simulink model "windSimulation_2020a"  (R2020a)
settings: Solver=ode4  StartTime=0.0  StopTime=100  FixedStep=dt  RelTol=1e-3
values from neighbouring files (symbols this model uses):
  alt0 = 600    [initializeSim.m]
  dt = 0.1    [dryden_wind_model.m]    (also in filters.m; full_sim_and_filter_loop.m = 0.01; getDynamicsJacobian.m; initializeSim.m = 0.01)
  F = [0;0;0]    [simple_sim.m]
  gustWindFlag = 1    [initializeSim.m]
  initCovarianceEkf = diag([1e-3, 1e-3,                            2, 5e-3,                            1e-4, 1e-4,                            10, 10])    [initializeSim.m]
  initCovarianceUKF = diag([1e-3, 1e-3,                            2, 5e-3,                            1e-4, 1e-4,                            1, 1])    [initializeSim.m]
  initEstimateEkf = [0, 0,                     initGroundSpeedEst, initAttitude(3),                     windNorthStatic + 4*randn, windEastStatic + 4*randn,                     0, 0]    [initializeSim.m]
  initEstimateParticleFilter = [0, 0, initGroundSpeedEst, initAttitude(3), 15, -32]    [initializeSim.m]
  initEstimateUKF = [0, 0, initGroundSpeedEst, initAttitude(3),                    windNorthStatic + 1*randn, windEastStatic + 1*randn,                     0, 0]    [initializeSim.m]
  q = uKF(2)    [dynJacobian.m]    (also in getDynamicsJacobian.m; getDynamicsJacobianTest.m; getStateTransitionDynamics.m; simple_sim.m)
  Qekf = diag([1e-5, 1e-5,               1, 1e-3,               1, 1,               1, 1])    [initializeSim.m]
  Qukf = diag([1e-5, 1e-5,               1, 1e-3,               .1, .1,               .1, .1])    [initializeSim.m]
  r = uKF(3)    [dynJacobian.m]    (also in getDynamicsJacobian.m; getDynamicsJacobianTest.m; getStateTransitionDynamics.m; simple_sim.m)
  Rekf = diag([1, 1,               1, 1e-3,               1, 1])    [initializeSim.m]
  Rukf = diag([1, 1,               1, 1e-3,               1, 1])    [initializeSim.m]
  sensorNoiseFlag = 1    [initializeSim.m]
  staticWindFlag = 1    [initializeSim.m]
  turbulentWindFlag = 1    [initializeSim.m]
  var = getSensorVariances('low')    [getSensorVariances.m]    (also in initializeSim.m = getSensorVariances(suite))
  windDownStatic = 0    [initializeSim.m]
  windEastStatic = -9    [initializeSim.m]
  windNorthStatic = 14    [initializeSim.m]
undefined symbols (not defined in the file or in its folder): MIL, sigbuilder_block
libraries: aerolibwind2 x2, shared6dof x1, sharedtransform x1, aerolibasang x1, simulink_extras x1
settings Model: Creator=Don  LastModifiedBy=Somrita

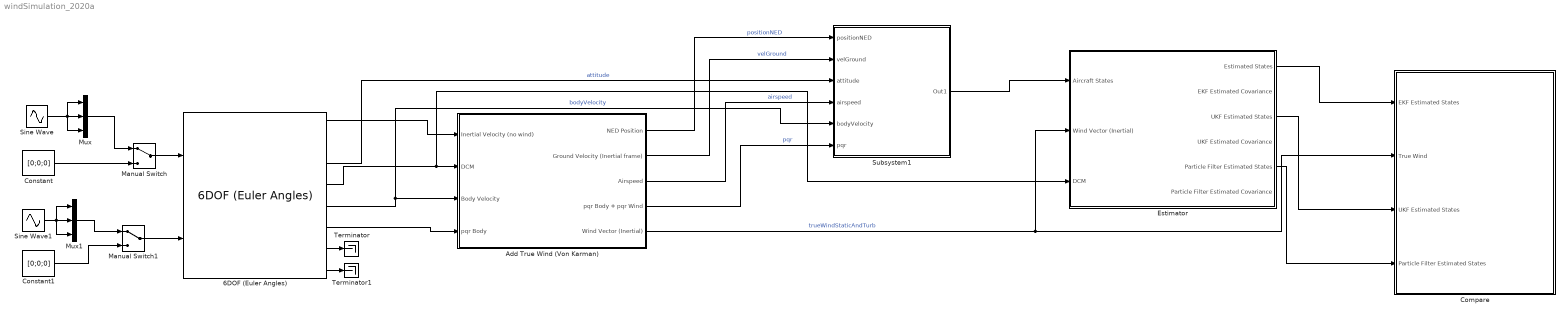
== system windSimulation_2020a ==
  6DOF (Euler Angles) : shared6dof/6DOF (Euler Angles)  units=Metric (MKS)  mtype=Fixed  rep=Euler Angles  xme_0=[0 0 -abs(alt0)]  Vm_0=initVelBody  eul_0=initAttitude  pm_0=[0 0 0]  mass_0=mass  mass_e=0.5  mass_f=2.0  inertia=J  inertia_e=eye(3)  inertia_f=2*eye(3)  k_quat=1.0  vre_flag=on  abi_flag=off  aMode=0  xme_statename=''  Vm_statename=''  eul_statename=''  quat_statename=''  pm_statename=''  mass_statename=''
      settings: SourceProductBaseCode=AE,PW,MT,UV,VE,VP
  Add True Wind (Von Karman) : Subsystem
  Compare : Subsystem
  Constant : Constant  Value=[0;0;0]
  Constant1 : Constant  Value=[0;0;0]
  Estimator : Subsystem
  Manual Switch : ManualSwitch
  Manual Switch1 : ManualSwitch
  Mux : Mux  Inputs=3
  Mux1 : Mux  Inputs=3
  Sine Wave : Sin  SampleTime=0
  Sine Wave1 : Sin  Amplitude=0.001  SampleTime=0
  Subsystem1 : Subsystem
  Terminator : Terminator
  Terminator1 : Terminator
  wires:
  Constant/1 -> Manual Switch/2
  Constant1/1 -> Manual Switch1/2
  6DOF (Euler Angles)/1 -> Add True Wind (Von Karman)/1(Inertial Velocity (no wind))
  6DOF (Euler Angles)/4 -> Estimator/3(DCM), Add True Wind (Von Karman)/2(DCM)
  6DOF (Euler Angles)/5 -> Add True Wind (Von Karman)/3(Body Velocity), Subsystem1/5(bodyVelocity)  "bodyVelocity"
  6DOF (Euler Angles)/6 -> Add True Wind (Von Karman)/4(pqr Body)
  Manual Switch/1 -> 6DOF (Euler Angles)/1
  Manual Switch1/1 -> 6DOF (Euler Angles)/2
  Sine Wave/1 -> Mux/2, Mux/1, Mux/3
  Mux/1 -> Manual Switch/1
  Sine Wave1/1 -> Mux1/2, Mux1/1, Mux1/3
  Mux1/1 -> Manual Switch1/1
  6DOF (Euler Angles)/7 -> Terminator/1
  6DOF (Euler Angles)/8 -> Terminator1/1
  Estimator/1(Estimated States) -> Compare/1(EKF Estimated States)
  Add True Wind (Von Karman)/5(Wind Vector (Inertial)) -> Estimator/2(Wind Vector (Inertial)), Compare/2(True Wind)  "trueWindStaticAndTurb"
  Estimator/3(UKF Estimated States) -> Compare/3(UKF Estimated States)
  Estimator/5(Particle Filter Estimated States) -> Compare/4(Particle Filter Estimated States)
  Add True Wind (Von Karman)/1(NED Position) -> Subsystem1/1(positionNED)  "positionNED"
  Add True Wind (Von Karman)/2(Ground Velocity (Inertial frame)) -> Subsystem1/2(velGround)  "velGround"
  6DOF (Euler Angles)/3 -> Subsystem1/3(attitude)  "attitude"
  Add True Wind (Von Karman)/3(Airspeed) -> Subsystem1/4(airspeed)  "airspeed"
  Add True Wind (Von Karman)/4(pqr Body + pqr Wind) -> Subsystem1/6(pqr)  "pqr"
  Subsystem1/1(Out1) -> Estimator/1(Aircraft States)

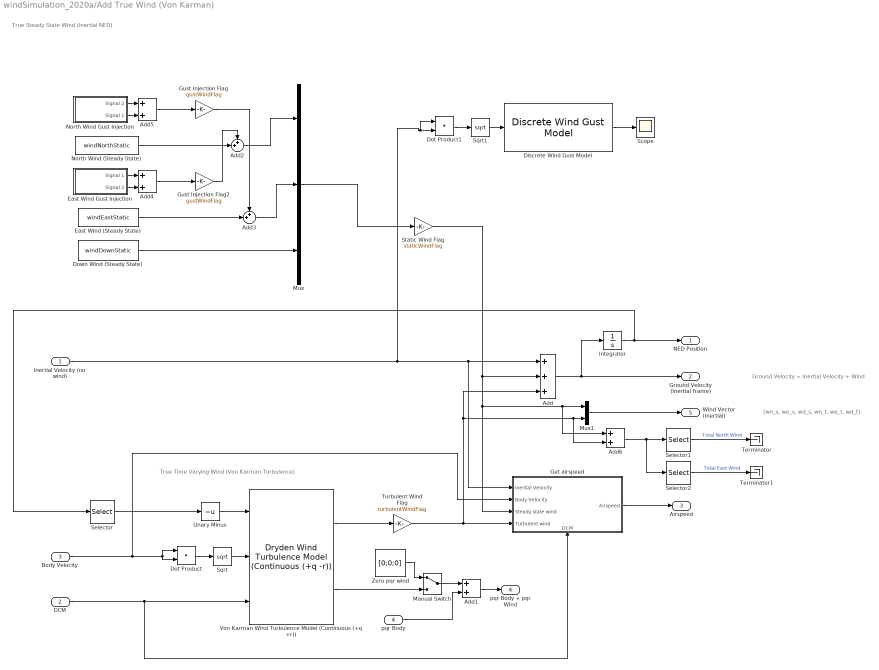
== system windSimulation_2020a/Add True Wind (Von Karman) ==
  note: [wn_s, we_s, wd_s, wn_t, we_t, wd_t]
  note: Ground Velocity = Inertial Velocity + Wind
  note: True Time Varying Wind (Von Karman Turbulence)
  note: True Steady State Wind (Inertial NED)
  Inertial Velocity (no wind) : Inport
  DCM : Inport  Port=2
  Body Velocity : Inport  Port=3
  pqr Body : Inport  Port=4
  Add : Sum  Inputs=+++
  Add{1,4..6} (4 alike) : Sum
  Add2 : Sum  Inputs=++|
  Add3 : Sum  Inputs=++|
  Discrete Wind Gust Model : aerolibwind2/Discrete Wind Gust Model  units=Metric (MKS)  Gx=on  Gy=on  Gz=on  t_0=5  d_m=[120 120 80]  v_m=[3.5 3.5 3.0]
  Dot Product : DotProduct  InputSameDT=on  OutDataTypeStr=Inherit: Inherit via internal rule
  Dot Product1 : DotProduct  InputSameDT=on  OutDataTypeStr=Inherit: Inherit via internal rule
  Down Wind (Steady State) : Constant  Value=windDownStatic
  East Wind (Steady State) : Constant  Value=windEastStatic
  East Wind Gust Injection : Subsystem  Tag=STV Subsys  LoadFcn=sigbuilder_block('load');  StartFcn=sigbuilder_block('start');  StopFcn=sigbuilder_block('stop');  ClipboardFcn=sigbuilder_block('clipboard');  mask(Sigbuilder block){tuvar=[0:10]}
      mask help: Simulink:masks:SigbuilderBlock_MD
      mask init:
      | if ~strcmp(get_param(bdroot(gcbh),'SimulationStatus'),'stopped') tuvar = sigbuilder_block('maskInit'); end
      settings: CopyFcn=sigbuilder_block('copy');  DeleteFcn=sigbuilder_block('delete');  ModelCloseFcn=sigbuilder_block('modelClose');  PreSaveFcn=sigbuilder_block('preSave');  PauseFcn=sigbuilder_block('pause');  ContinueFcn=sigbuilder_block('continue');  NameChangeFcn=sigbuilder_block('namechange');  OpenFcn=sigbuilder_block('open',[48.75 0 1391.25 750.75 ]);  CloseFcn=sigbuilder_block('close');
      mask Display: plot(0, 0, 100, 100,[2, 2, 32, 32, 2], [68, 8, 8, 68, 68],[32, 2], [38, 38], [32, 19, 2],[53, 60, 44], [32, 17, 17, 2],[16, 16, 31, 31]);txt = getActiveGroup(gcbh);text(2, 100, txt,'verticalAlignment', 'top');
  Get airspeed : Subsystem
      settings: PortSchema="{\"entries\":[{\"content\":{\"sides\":[{\"content\":{\"connectorIds\":[\"In1\",\"In2\",\"In3\",\"In4\"]},\"type\":\"ConnectorPlacement.EquallySpacedRectSide\",\"uuid\":\"813c2b5b-04f3-4ec3-a969-2504c20ca38b\"},{\"content\":{\"connectorIds\":[\"Out1\"],\"side\":\"RIGHT\"},\"type\":\"ConnectorPlacement.EquallySpacedRectSide\",\"uuid\":\"9f878792-4dd4-4000-acee-7f28349bdd5f\"},{\"content\":{\"connectorIds\":[],\"side\":\"TOP\"},\"type\":\"ConnectorPlacement.EquallySpacedRectSide\",\"uuid\":\"3d2ef613-18a7-4015-9ddb-8a03be605fb8\"},{\"content\":{\"connectorIds\":[\"In5\"],\"side\":\"BOTTOM\"},\"type\":\"ConnectorPlacement.EquallySpacedRectSide\",\"uuid\":\"121bcea6-4847-4a17-8a68-e62f0e126d50\"}]},\"type\":\"ConnectorPlacement.EquallySpacedConnector\",\"uuid\":\"0bfc4666-1d36-45c8-946f-537367ff2a54\"}],\"packageUris\":[\"http://schema.mathworks.com/mf0/Connector/19700101\"],\"version\":\"1.0\"}"
  Gust Injection Flag : Gain  Gain=gustWindFlag
  Gust Injection Flag2 : Gain  Gain=gustWindFlag
  Integrator : Integrator  InitialCondition=[0, 0, -abs(alt0)]
  Manual Switch : ManualSwitch
  Mux : Mux  Inputs=3
  Mux1 : Mux  Inputs=2
  North Wind (Steady State) : Constant  Value=windNorthStatic
  North Wind Gust Injection : Subsystem  Tag=STV Subsys  LoadFcn=sigbuilder_block('load');  StartFcn=sigbuilder_block('start');  StopFcn=sigbuilder_block('stop');  ClipboardFcn=sigbuilder_block('clipboard');  mask(Sigbuilder block){tuvar=[0:10]}
      mask help: Simulink:masks:SigbuilderBlock_MD
      mask init:
      | if ~strcmp(get_param(bdroot(gcbh),'SimulationStatus'),'stopped') tuvar = sigbuilder_block('maskInit'); end
      settings: CopyFcn=sigbuilder_block('copy');  DeleteFcn=sigbuilder_block('delete');  ModelCloseFcn=sigbuilder_block('modelClose');  PreSaveFcn=sigbuilder_block('preSave');  PauseFcn=sigbuilder_block('pause');  ContinueFcn=sigbuilder_block('continue');  NameChangeFcn=sigbuilder_block('namechange');  OpenFcn=sigbuilder_block('open',[48.75 0 1391.25 729.75 ]);  CloseFcn=sigbuilder_block('close');
      mask Display: plot(0, 0, 100, 100,[2, 2, 32, 32, 2], [68, 8, 8, 68, 68],[32, 2], [38, 38], [32, 19, 2],[53, 60, 44], [32, 17, 17, 2],[16, 16, 31, 31]);txt = getActiveGroup(gcbh);text(2, 100, txt,'verticalAlignment', 'top');
  Scope : Scope
  Selector : Selector  InputPortWidth=3  IndexOptions=Index vector (dialog)  Indices=3  OutputSizes=1
  Selector1 : Selector  InputPortWidth=3  IndexOptions=Index vector (dialog)  Indices=1  OutputSizes=1
  Selector2 : Selector  InputPortWidth=3  IndexOptions=Index vector (dialog)  Indices=2  OutputSizes=1
  Sqrt : Sqrt  SaturateOnIntegerOverflow=on
  Sqrt1 : Sqrt  SaturateOnIntegerOverflow=on
  Static Wind Flag : Gain  Gain=staticWindFlag
  Terminator : Terminator
  Terminator1 : Terminator
  Turbulent Wind Flag : Gain  Gain=turbulentWindFlag
  Unary Minus : UnaryMinus
  Von Karman Wind Turbulence Model (Continuous (+q +r)) : aerolibwind2/Dryden Wind Turbulence Model  (Continuous (+q -r))  units=Metric (MKS)  spec=MIL-F-8785C  model=Continuous Von Karman (+q +r)  W20=10  Wdeg=0  TurbProb=10^-1  L_high=762  Wingspan=10  ts=0.1  Seed=[23341 23342 23343 23344]  T_on=on
  Zero pqr wind : Constant  Value=[0;0;0]
  NED Position : Outport  PortDimensions=3
  Ground Velocity (Inertial frame) : Outport  Port=2
  Airspeed : Outport  Port=3  PortDimensions=1
  pqr Body + pqr Wind : Outport  Port=4
  Wind Vector (Inertial) : Outport  Port=5
  wires:
  Sqrt/1 -> Von Karman Wind Turbulence Model (Continuous (+q +r))/2
  Selector/1 -> Unary Minus/1
  Von Karman Wind Turbulence Model (Continuous (+q +r))/1 -> Turbulent Wind Flag/1
  Unary Minus/1 -> Von Karman Wind Turbulence Model (Continuous (+q +r))/1
  DCM/1 -> Get airspeed/5(DCM), Von Karman Wind Turbulence Model (Continuous (+q +r))/3
  Body Velocity/1 -> Get airspeed/2(Body Velocity), Dot Product/2, Dot Product/1
  Von Karman Wind Turbulence Model (Continuous (+q +r))/2 -> Manual Switch/2
  Add/1 -> Ground Velocity (Inertial frame)/1, Integrator/1
  Add1/1 -> pqr Body + pqr Wind/1
  pqr Body/1 -> Add1/2
  North Wind (Steady State)/1 -> Add2/2
  East Wind (Steady State)/1 -> Add3/2
  Down Wind (Steady State)/1 -> Mux/3
  Mux/1 -> Static Wind Flag/1
  Manual Switch/1 -> Add1/1
  Zero pqr wind/1 -> Manual Switch/1
  Get airspeed/1(Airspeed) -> Airspeed/1
  Dot Product/1 -> Sqrt/1
  Mux1/1 -> Wind Vector (Inertial)/1
  Integrator/1 -> Selector/1, NED Position/1
  Turbulent Wind Flag/1 -> Get airspeed/4(Turbulent wind), Add/3, Add6/2, Mux1/2
  Static Wind Flag/1 -> Add6/1, Mux1/1, Get airspeed/3(Steady state wind), Add/2
  Add3/1 -> Mux/2
  Add2/1 -> Mux/1
  East Wind Gust Injection/1(Signal 1) -> Add4/1
  East Wind Gust Injection/2(Signal 2) -> Add4/2
  Add4/1 -> Gust Injection Flag2/1
  Add5/1 -> Gust Injection Flag/1
  North Wind Gust Injection/1(Signal 2) -> Add5/1
  North Wind Gust Injection/2(Signal 1) -> Add5/2
  Gust Injection Flag/1 -> Add3/1
  Gust Injection Flag2/1 -> Add2/1
  Sqrt1/1 -> Discrete Wind Gust Model/1
  Dot Product1/1 -> Sqrt1/1
  Inertial Velocity (no wind)/1 -> Dot Product1/1, Dot Product1/2, Get airspeed/1(Inertial Velocity), Add/1
  Discrete Wind Gust Model/1 -> Scope/1
  Add6/1 -> Selector2/1, Selector1/1
  Selector1/1 -> Terminator/1  "Total North Wind"
  Selector2/1 -> Terminator1/1  "Total East Wind"

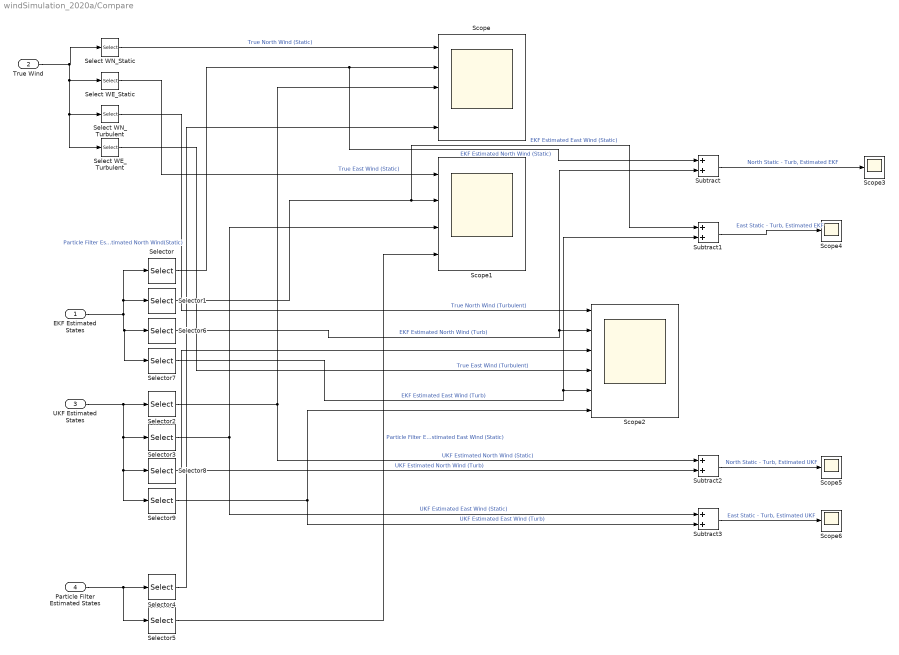
== system windSimulation_2020a/Compare ==
  EKF Estimated States : Inport
  True Wind : Inport  Port=2
  UKF Estimated States : Inport  Port=3
  Particle Filter Estimated States : Inport  Port=4
  Scope : Scope  NumInputPorts=5
  Scope1 : Scope  NumInputPorts=4
  Scope2 : Scope  NumInputPorts=6
  Scope{3..6} (4 alike) : Scope
  Select WE_Static : Selector  InputPortWidth=6  IndexOptions=Index vector (dialog)  Indices=2  OutputSizes=1
  Select WE_Turbulent : Selector  InputPortWidth=6  IndexOptions=Index vector (dialog)  Indices=5  OutputSizes=1
  Select WN_Static : Selector  InputPortWidth=6  IndexOptions=Index vector (dialog)  Indices=1  OutputSizes=1
  Select WN_Turbulent : Selector  InputPortWidth=6  IndexOptions=Index vector (dialog)  Indices=4  OutputSizes=1
  Selector : Selector  InputPortWidth=nEstStates  IndexOptions=Index vector (dialog)  Indices=5  OutputSizes=1
  Selector1 : Selector  InputPortWidth=nEstStates  IndexOptions=Index vector (dialog)  Indices=6  OutputSizes=1
  Selector2 : Selector  InputPortWidth=nEstStates  IndexOptions=Index vector (dialog)  Indices=5  OutputSizes=1
  Selector3 : Selector  InputPortWidth=nEstStates  IndexOptions=Index vector (dialog)  Indices=6  OutputSizes=1
  Selector4 : Selector  InputPortWidth=nEstStates  IndexOptions=Index vector (dialog)  Indices=5  OutputSizes=1
  Selector5 : Selector  InputPortWidth=nEstStates  IndexOptions=Index vector (dialog)  Indices=6  OutputSizes=1
  Selector6 : Selector  InputPortWidth=nEstStates  IndexOptions=Index vector (dialog)  Indices=7  OutputSizes=1
  Selector7 : Selector  InputPortWidth=nEstStates  IndexOptions=Index vector (dialog)  Indices=8  OutputSizes=1
  Selector8 : Selector  InputPortWidth=nEstStates  IndexOptions=Index vector (dialog)  Indices=7  OutputSizes=1
  Selector9 : Selector  InputPortWidth=nEstStates  IndexOptions=Index vector (dialog)  Indices=8  OutputSizes=1
  Subtract{,1..3} (4 alike) : Sum
  wires:
  EKF Estimated States/1 -> Selector7/1, Selector6/1, Selector1/1, Selector/1
  True Wind/1 -> Select WE_Turbulent/1, Select WN_Turbulent/1, Select WE_Static/1, Select WN_Static/1
  Selector/1 -> Subtract/1, Scope/2  "EKF Estimated North Wind (Static)"
  Select WN_Static/1 -> Scope/1  "True North Wind (Static)"
  Selector1/1 -> Subtract1/1, Scope1/2  "EKF Estimated East Wind (Static)"
  Select WE_Static/1 -> Scope1/1  "True East Wind (Static)"
  UKF Estimated States/1 -> Selector9/1, Selector8/1, Selector3/1, Selector2/1
  Selector2/1 -> Scope/3, Subtract2/1  "UKF Estimated North Wind (Static)"
  Selector3/1 -> Scope1/3, Subtract3/1  "UKF Estimated East Wind (Static)"
  Particle Filter Estimated States/1 -> Selector5/1, Selector4/1
  Selector4/1 -> Scope/5  "Particle Filter Estimated North Wind(Static)"
  Selector5/1 -> Scope1/4  "Particle Filter Estimated East Wind (Static)"
  Selector6/1 -> Subtract/2, Scope2/2  "EKF Estimated North Wind (Turb)"
  Selector7/1 -> Subtract1/2, Scope2/5  "EKF Estimated East Wind (Turb)"
  Select WN_Turbulent/1 -> Scope2/1  "True North Wind (Turbulent)"
  Select WE_Turbulent/1 -> Scope2/4  "True East Wind (Turbulent)"
  Subtract/1 -> Scope3/1  "North Static - Turb, Estimated EKF"
  Subtract1/1 -> Scope4/1  "East Static - Turb, Estimated EKF"
  Selector8/1 -> Subtract2/2, Scope2/3  "UKF Estimated North Wind (Turb)"
  Selector9/1 -> Subtract3/2, Scope2/6  "UKF Estimated East Wind (Turb)"
  Subtract3/1 -> Scope6/1  "East Static - Turb, Estimated UKF"
  Subtract2/1 -> Scope5/1  "North Static - Turb, Estimated UKF"

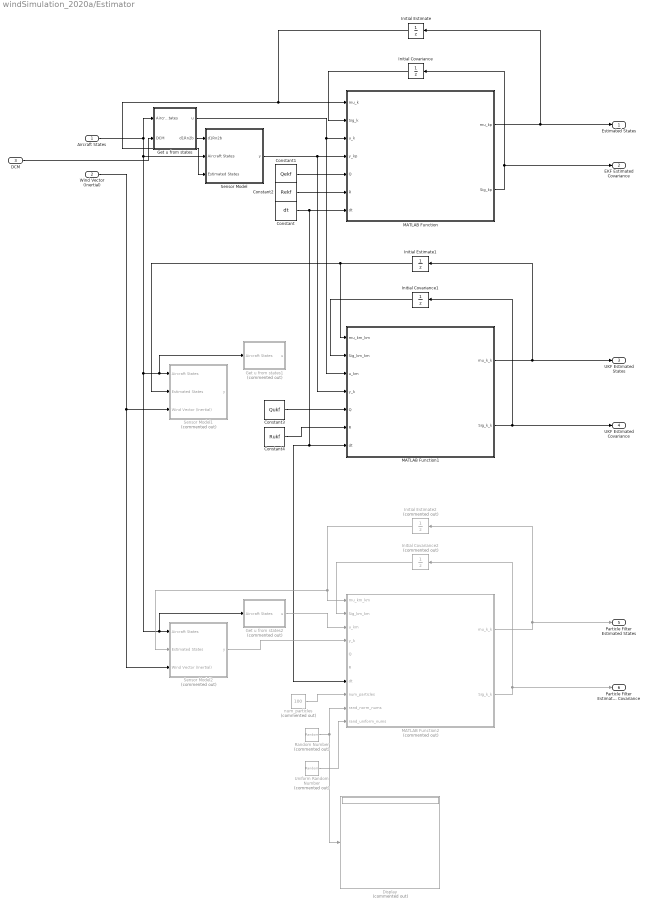
== system windSimulation_2020a/Estimator ==
  Aircraft States : Inport
  Wind Vector (Inertial) : Inport  Port=2
  DCM : Inport  Port=3
  Constant : Constant  Value=dt
  Constant1 : Constant  Value=Qekf
  Constant2 : Constant  Value=Rekf
  Constant3 : Constant  Value=Qukf
  Constant4 : Constant  Value=Rukf
  Display : Display  Commented=on
  Get u from states : Subsystem
  Get u from states1 : Subsystem  Commented=on
  Get u from states2 : Subsystem  Commented=on
  Initial Covariance : UnitDelay  InitialCondition=initCovarianceEkf  SampleTime=-1  HasFrameUpgradeWarning=on
  Initial Covariance1 : UnitDelay  InitialCondition=initCovarianceUKF  SampleTime=-1  HasFrameUpgradeWarning=on
  Initial Covariance2 : UnitDelay  Commented=on  InitialCondition=initCovarianceEkf  SampleTime=-1  HasFrameUpgradeWarning=on
  Initial Estimate : UnitDelay  InitialCondition=initEstimateEkf  SampleTime=-1  HasFrameUpgradeWarning=on
  Initial Estimate1 : UnitDelay  InitialCondition=initEstimateUKF  SampleTime=-1  HasFrameUpgradeWarning=on
  Initial Estimate2 : UnitDelay  Commented=on  InitialCondition=initEstimateParticleFilter  SampleTime=-1  HasFrameUpgradeWarning=on
  MATLAB Function : MATLAB Function  TreatAsAtomicUnit=on
  MATLAB Function1 : MATLAB Function  TreatAsAtomicUnit=on
  MATLAB Function2 : MATLAB Function  Commented=on  TreatAsAtomicUnit=on
  Random Number : RandomNumber  Commented=on  Mean=zeros(100*6,1)  Seed=1:6*100  SampleTime=0.1
  Sensor Model : Subsystem
  Sensor Model1 : Subsystem  Commented=on
  Sensor Model2 : Subsystem  Commented=on
  Uniform Random Number : UniformRandomNumber  Commented=on  Minimum=zeros(100,1)  Maximum=ones(100,1)  Seed=1:100  SampleTime=0.1
  num_particles : Constant  Commented=on  Value=100
  Estimated States : Outport
  EKF Estimated Covariance : Outport  Port=2
  UKF Estimated States : Outport  Port=3
  UKF Estimated Covariance : Outport  Port=4
  Particle Filter Estimated States : Outport  Port=5
  Particle Filter Estimated Covariance : Outport  Port=6
  wires:
  MATLAB Function/1(mu_kp) -> Initial Estimate/1, Estimated States/1
  Initial Estimate/1 -> Sensor Model/3(Estimated States), MATLAB Function/1(mu_k)
  MATLAB Function/2(Sig_kp) -> EKF Estimated Covariance/1, Initial Covariance/1
  Initial Covariance/1 -> MATLAB Function/2(Sig_k)
  MATLAB Function1/1(mu_k_k) -> UKF Estimated States/1, Initial Estimate1/1
  MATLAB Function1/2(Sig_k_k) -> UKF Estimated Covariance/1, Initial Covariance1/1
  Initial Estimate1/1 -> MATLAB Function1/1(mu_km_km), Sensor Model1/2(Estimated States)
  Initial Covariance1/1 -> MATLAB Function1/2(Sig_km_km)
  MATLAB Function2/1(mu_k_k) -> Particle Filter Estimated States/1, Initial Estimate2/1
  Constant/1 -> MATLAB Function2/7(dt), MATLAB Function1/7(dt), MATLAB Function/7(dt)
  Sensor Model/1(y) -> MATLAB Function1/4(y_k), MATLAB Function/4(y_kp)
  MATLAB Function2/2(Sig_k_k) -> Particle Filter Estimated Covariance/1, Initial Covariance2/1
  Constant2/1 -> MATLAB Function/6(R)
  Constant1/1 -> MATLAB Function/5(Q)
  Initial Covariance2/1 -> MATLAB Function2/2(Sig_km_km)
  Get u from states/1(u) -> MATLAB Function1/3(u_km), MATLAB Function/3(u_k)
  Random Number/1 -> Display/1, MATLAB Function2/9(rand_norm_nums)
  num_particles/1 -> MATLAB Function2/8(num_particles)
  Uniform Random Number/1 -> MATLAB Function2/10(rand_uniform_nums)
  Wind Vector (Inertial)/1 -> Sensor Model2/3(Wind Vector (Inertial)), Sensor Model1/3(Wind Vector (Inertial))
  Aircraft States/1 -> Sensor Model2/1(Aircraft States), Get u from states2/1(Aircraft States), Sensor Model1/1(Aircraft States), Get u from states1/1(Aircraft States), Sensor Model/2(Aircraft States), Get u from states/1(Aircraft States)
  Initial Estimate2/1 -> MATLAB Function2/1(mu_km_km), Sensor Model2/2(Estimated States)
  Get u from states2/1(u) -> MATLAB Function2/3(u_km)
  Sensor Model2/1(y) -> MATLAB Function2/4(y_k)
  Constant3/1 -> MATLAB Function1/5(Q)
  Constant4/1 -> MATLAB Function1/6(R)
  Get u from states/2(d1Rn2b) -> Sensor Model/1(d1Rn2b)
  DCM/1 -> Get u from states/2(DCM)

== system windSimulation_2020a/Subsystem1 ==
  note: xyzInertial, uvwGround, attitude, pqr, airspeed, groundSpeed, courseAngle
  positionNED : Inport
  velGround : Inport  Port=2
  attitude : Inport  Port=3
  airspeed : Inport  Port=4
  bodyVelocity : Inport  Port=5
  pqr : Inport  Port=6
  Get ground speed and course angle : Subsystem
  Mux2 : Mux  Inputs=8
  Subsystem : Subsystem
  Out1 : Outport
  wires:
  positionNED/1 -> Mux2/1
  airspeed/1 -> Mux2/5
  Subsystem/1(Aligned Attitude) -> Mux2/3
  bodyVelocity/1 -> Mux2/8, Subsystem/2(bodyVelocity)
  attitude/1 -> Subsystem/1(Attitude)
  Get ground speed and course angle/1(Ground Speed) -> Mux2/6  "trueGroundspeed"
  Get ground speed and course angle/2(Course Angle) -> Mux2/7  "trueCourseAngle"
  velGround/1 -> Mux2/2, Get ground speed and course angle/1(Ground Velocity)
  Mux2/1 -> Out1/1
  pqr/1 -> Mux2/4

== system windSimulation_2020a/Add True Wind (Von Karman)/East Wind Gust Injection ==
  Demux : Demux  Tag=STV Demux  Outputs=2
      settings: DisplayOption=none
  FromWs : FromWorkspace  Tag=STV FromWs  VariableName=tuvar
      SigBuilderData=|
      | common.afterFinalStr = 'Extrapolate'
      | common.sampleTime = 0
      | dataSet.timeRange = [0 100]
      | dataSet.name = 'Group 1'
      | sbobj.Groups.Name = 'Group 1'
      | sbobj.Groups.Signals(1).Name = 'Signal 1'
      | sbobj.Groups.Signals(1).XData = [0 6 6 18 18 100]
      | sbobj.Groups.Signals(1).YData = [0 0 7 7 0 0]
      | sbobj.Groups.Signals(2).Name = 'Signal 2'
      | sbobj.Groups.Signals(2).XData = [0 42 42 58 58 100]
      | sbobj.Groups.Signals(2).YData = [0 0 -3 -3 0 0]
      | sbobj.Groups.TimeRange = [0 100]
  Signal 1 : Outport  Tag=STV Outport
  Signal 2 : Outport  Tag=STV Outport  Port=2
  wires:
  FromWs/1 -> Demux/1
  Demux/1 -> Signal 1/1
  Demux/2 -> Signal 2/1

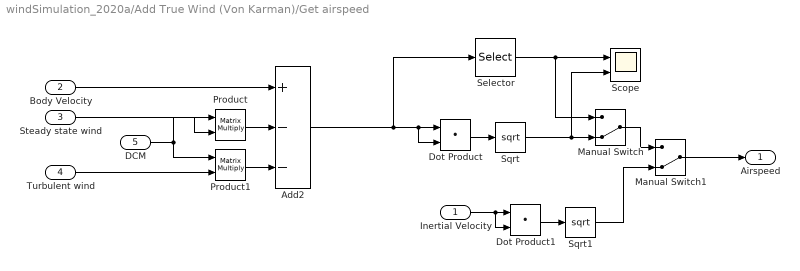
== system windSimulation_2020a/Add True Wind (Von Karman)/Get airspeed ==
  Inertial Velocity : Inport
  Body Velocity : Inport  Port=2
  Steady state wind : Inport  Port=3
  Turbulent wind : Inport  Port=4
  DCM : Inport  Port=5
  Add2 : Sum  Inputs=+--
  Dot Product : DotProduct  InputSameDT=on  OutDataTypeStr=Inherit: Inherit via internal rule
  Dot Product1 : DotProduct  InputSameDT=on  OutDataTypeStr=Inherit: Inherit via internal rule
  Manual Switch : ManualSwitch  CurrentSetting=0
  Manual Switch1 : ManualSwitch  CurrentSetting=0
  Product : Product  Multiplication=Matrix(*)
  Product1 : Product  Multiplication=Matrix(*)
  Scope : Scope  NumInputPorts=2
  Selector : Selector  InputPortWidth=3  IndexOptions=Index vector (dialog)  Indices=1  OutputSizes=1
  Sqrt : Sqrt  SaturateOnIntegerOverflow=on
  Sqrt1 : Sqrt  SaturateOnIntegerOverflow=on
  Airspeed : Outport
  wires:
  Body Velocity/1 -> Add2/1
  Steady state wind/1 -> Product/2
  Add2/1 -> Dot Product/2, Dot Product/1, Selector/1
  Turbulent wind/1 -> Product1/2
  DCM/1 -> Product/1, Product1/1
  Product/1 -> Add2/2
  Product1/1 -> Add2/3
  Manual Switch/1 -> Manual Switch1/1
  Selector/1 -> Manual Switch/1, Scope/1
  Dot Product/1 -> Sqrt/1
  Sqrt/1 -> Scope/2, Manual Switch/2
  Manual Switch1/1 -> Airspeed/1
  Dot Product1/1 -> Sqrt1/1
  Inertial Velocity/1 -> Dot Product1/1, Dot Product1/2
  Sqrt1/1 -> Manual Switch1/2

== system windSimulation_2020a/Add True Wind (Von Karman)/North Wind Gust Injection ==
  Demux : Demux  Tag=STV Demux  Outputs=2
      settings: DisplayOption=none
  FromWs : FromWorkspace  Tag=STV FromWs  VariableName=tuvar
      SigBuilderData=|
      | common.afterFinalStr = 'Extrapolate'
      | common.sampleTime = 0
      | dataSet.timeRange = [0 100]
      | dataSet.name = 'Group 1'
      | sbobj.Groups.Name = 'Group 1'
      | sbobj.Groups.Signals(1).Name = 'Signal 2'
      | sbobj.Groups.Signals(1).XData = [0 52 52 69 69.1 100]
      | sbobj.Groups.Signals(1).YData = [0 0 6 6 0 0]
      | sbobj.Groups.Signals(2).Name = 'Signal 1'
      | sbobj.Groups.Signals(2).XData = [0 8 8 23 23 100]
      | sbobj.Groups.Signals(2).YData = [0 0 -4 -4 0 0]
      | sbobj.Groups.TimeRange = [0 100]
  Signal 2 : Outport  Tag=STV Outport
  Signal 1 : Outport  Tag=STV Outport  Port=2
  wires:
  FromWs/1 -> Demux/1
  Demux/1 -> Signal 2/1
  Demux/2 -> Signal 1/1

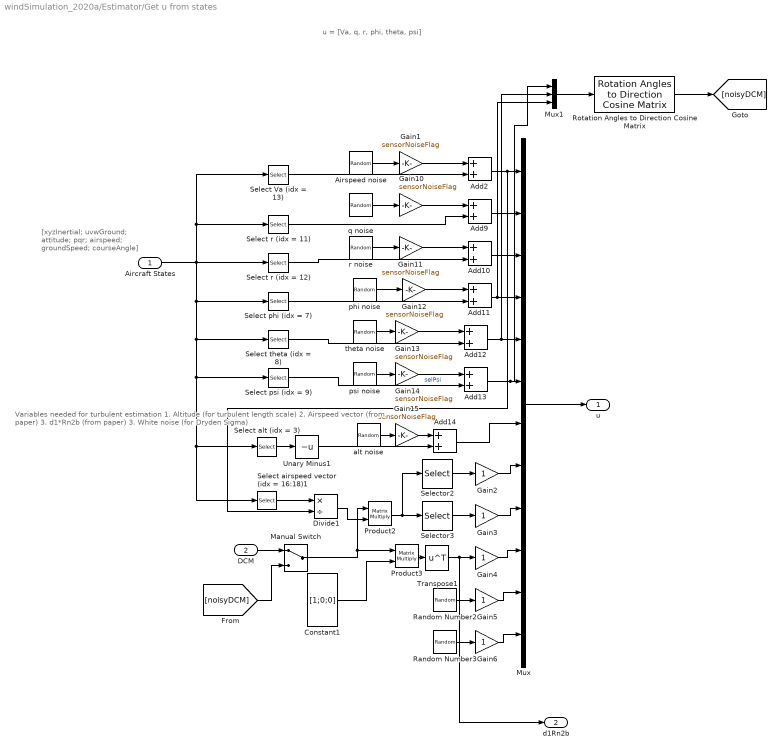
== system windSimulation_2020a/Estimator/Get u from states ==
  note: Variables needed for turbulent estimation
      | 	1. Altitude (for turbulent length scale)
      | 	2. Airspeed vector (from paper)
      | 	3. d1*Rn2b (from paper)
      | 	3. White noise (for Dryden Sigma)
  note: u = [Va, q, r, phi, theta, psi]
  note: [xyzInertial;
      | uvwGround;
      | attitude;
      | pqr;
      | airspeed;
      | groundSpeed;
      | courseAngle]
  Aircraft States : Inport
  DCM : Inport  Port=2
  Add{2,9..14} (7 alike) : Sum
  Airspeed noise : RandomNumber  Variance=var.airspeed_mps  SampleTime=dt
  Constant1 : Constant  Value=[1;0;0]  VectorParams1D=off
  Divide1 : Product  Inputs=*/
  Gain{1,10..15} (7 alike) : Gain  Gain=sensorNoiseFlag
  Gain{2..6} (5 alike) : Gain
  Manual Switch : ManualSwitch
  Mux : Mux  Inputs=12
  Mux1 : Mux  Inputs=3
  Product2 : Product  Multiplication=Matrix(*)
  Product3 : Product  Multiplication=Matrix(*)
  Random Number2 : RandomNumber  SampleTime=dt
  Random Number3 : RandomNumber  Seed=100  SampleTime=dt
  Rotation Angles to Direction Cosine Matrix : sharedtransform/Rotation Angles to Direction Cosine Matrix  rotationOrder=ZYX  aMode=aMode
      settings: SourceProductBaseCode=AE,PW,MT,UV,VE,VP
  Select Va (idx = 13) : Selector  InputPortWidth=nStates  IndexOptions=Index vector (dialog)  Indices=13  OutputSizes=1
  Select airspeed vector (idx = 16:18)1 : Selector  InputPortWidth=nStates  IndexOptions=Index vector (dialog)  Indices=[16:18]  OutputSizes=1
  Select alt (idx = 3) : Selector  InputPortWidth=nStates  IndexOptions=Index vector (dialog)  Indices=3  OutputSizes=1
  Select phi (idx = 7) : Selector  InputPortWidth=nStates  IndexOptions=Index vector (dialog)  Indices=7  OutputSizes=1
  Select psi (idx = 9) : Selector  InputPortWidth=nStates  IndexOptions=Index vector (dialog)  Indices=9  OutputSizes=1
  Select r (idx = 11) : Selector  InputPortWidth=nStates  IndexOptions=Index vector (dialog)  Indices=11  OutputSizes=1
  Select r (idx = 12) : Selector  InputPortWidth=nStates  IndexOptions=Index vector (dialog)  Indices=12  OutputSizes=1
  Select theta (idx = 8) : Selector  InputPortWidth=nStates  IndexOptions=Index vector (dialog)  Indices=8  OutputSizes=1
  Selector2 : Selector  InputPortWidth=3  IndexOptions=Index vector (dialog)  Indices=1  OutputSizes=1
  Selector3 : Selector  InputPortWidth=3  IndexOptions=Index vector (dialog)  Indices=2  OutputSizes=1
  Transpose1 : Math  Operator=transpose  SaturateOnIntegerOverflow=on
  Unary Minus1 : UnaryMinus
  alt noise : RandomNumber  Variance=var.altitude_m  SampleTime=dt
  phi noise : RandomNumber  Variance=var.attitude_rad  SampleTime=dt
  psi noise : RandomNumber  Variance=var.attitude_rad * 3  SampleTime=dt
  q noise : RandomNumber  Variance=var.pqr_radps  SampleTime=dt
  r noise : RandomNumber  Variance=var.pqr_radps  SampleTime=dt
  theta noise : RandomNumber  Variance=var.attitude_rad  SampleTime=dt
  u : Outport
  d1Rn2b : Outport  Port=2
  wires:
  Aircraft States/1 -> Select airspeed vector (idx = 16:18)1/1, Select alt (idx = 3)/1, Select psi (idx = 9)/1, Select theta (idx = 8)/1, Select phi (idx = 7)/1, Select r (idx = 12)/1, Select r (idx = 11)/1, Select Va (idx = 13)/1
  Mux/1 -> u/1
  Select Va (idx = 13)/1 -> Add2/2
  Gain1/1 -> Add2/1
  Airspeed noise/1 -> Gain1/1
  Add2/1 -> Divide1/2, Mux/1
  q noise/1 -> Gain10/1
  Gain15/1 -> Add14/1
  Add9/1 -> Mux/2
  Add11/1 -> Mux1/3, Mux/4
  Add13/1 -> Mux1/1, Mux/6
  Add12/1 -> Mux1/2, Mux/5
  alt noise/1 -> Gain15/1
  Gain14/1 -> Add13/1
  theta noise/1 -> Gain13/1
  Add10/1 -> Mux/3
  r noise/1 -> Gain11/1
  Gain12/1 -> Add11/1
  Gain11/1 -> Add10/1
  psi noise/1 -> Gain14/1
  Gain13/1 -> Add12/1
  Gain10/1 -> Add9/1
  phi noise/1 -> Gain12/1
  Select r (idx = 11)/1 -> Add9/2
  Select r (idx = 12)/1 -> Add10/2
  Select phi (idx = 7)/1 -> Add11/2
  Select theta (idx = 8)/1 -> Add12/2
  Select psi (idx = 9)/1 -> Add13/2  "selPsi"
  Select alt (idx = 3)/1 -> Unary Minus1/1
  Unary Minus1/1 -> Add14/2
  Select airspeed vector (idx = 16:18)1/1 -> Divide1/1
  Divide1/1 -> Product2/2
  Selector2/1 -> Gain2/1
  Selector3/1 -> Gain3/1
  Product2/1 -> Selector2/1, Selector3/1
  Gain2/1 -> Mux/8
  Gain3/1 -> Mux/9
  Transpose1/1 -> d1Rn2b/1, Gain4/1
  Product3/1 -> Transpose1/1
  Constant1/1 -> Product3/2
  Random Number2/1 -> Gain5/1
  Random Number3/1 -> Gain6/1
  Gain4/1 -> Mux/10
  Gain5/1 -> Mux/11
  Gain6/1 -> Mux/12
  Add14/1 -> Mux/7
  Mux1/1 -> Rotation Angles to Direction Cosine Matrix/1
  Rotation Angles to Direction Cosine Matrix/1 -> [noisyDCM]
  [noisyDCM] -> Manual Switch/2
  Manual Switch/1 -> Product2/1, Product3/1
  DCM/1 -> Manual Switch/1

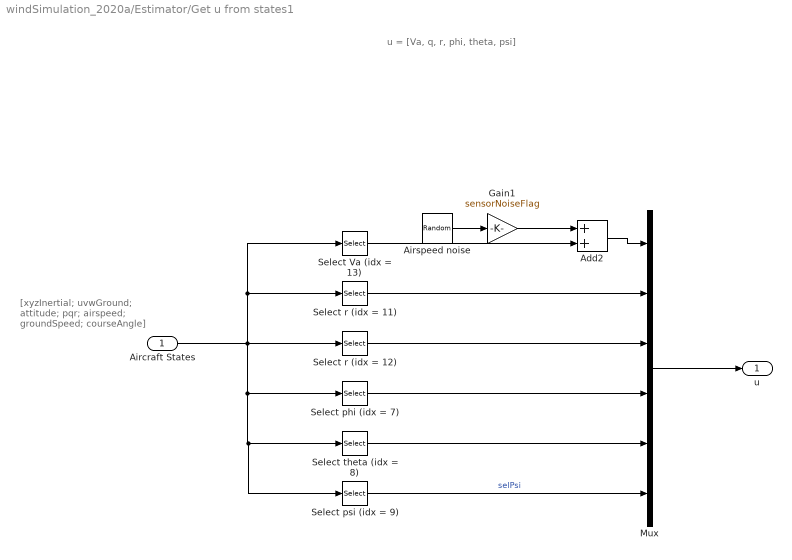
== system windSimulation_2020a/Estimator/Get u from states1 ==
  note: u = [Va, q, r, phi, theta, psi]
  note: [xyzInertial;
      | uvwGround;
      | attitude;
      | pqr;
      | airspeed;
      | groundSpeed;
      | courseAngle]
  Aircraft States : Inport
  Add2 : Sum
  Airspeed noise : RandomNumber  SampleTime=0.1
  Gain1 : Gain  Gain=sensorNoiseFlag
  Mux : Mux  Inputs=6
  Select Va (idx = 13) : Selector  InputPortWidth=15  IndexOptions=Index vector (dialog)  Indices=13  OutputSizes=1
  Select phi (idx = 7) : Selector  InputPortWidth=15  IndexOptions=Index vector (dialog)  Indices=7  OutputSizes=1
  Select psi (idx = 9) : Selector  InputPortWidth=15  IndexOptions=Index vector (dialog)  Indices=9  OutputSizes=1
  Select r (idx = 11) : Selector  InputPortWidth=15  IndexOptions=Index vector (dialog)  Indices=11  OutputSizes=1
  Select r (idx = 12) : Selector  InputPortWidth=15  IndexOptions=Index vector (dialog)  Indices=12  OutputSizes=1
  Select theta (idx = 8) : Selector  InputPortWidth=15  IndexOptions=Index vector (dialog)  Indices=8  OutputSizes=1
  u : Outport
  wires:
  Aircraft States/1 -> Select psi (idx = 9)/1, Select theta (idx = 8)/1, Select phi (idx = 7)/1, Select r (idx = 12)/1, Select r (idx = 11)/1, Select Va (idx = 13)/1
  Mux/1 -> u/1
  Select r (idx = 11)/1 -> Mux/2
  Select Va (idx = 13)/1 -> Add2/2
  Select r (idx = 12)/1 -> Mux/3
  Select phi (idx = 7)/1 -> Mux/4
  Select theta (idx = 8)/1 -> Mux/5
  Select psi (idx = 9)/1 -> Mux/6  "selPsi"
  Gain1/1 -> Add2/1
  Airspeed noise/1 -> Gain1/1
  Add2/1 -> Mux/1

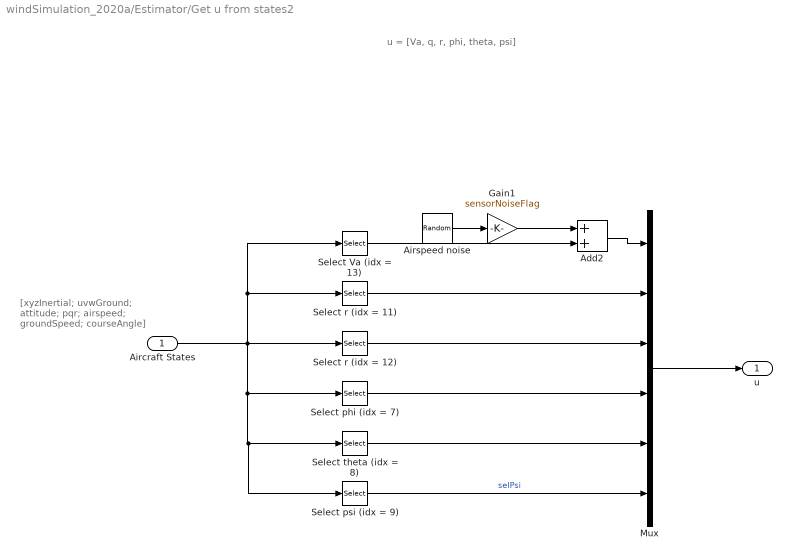
== system windSimulation_2020a/Estimator/Get u from states2 ==
  note: u = [Va, q, r, phi, theta, psi]
  note: [xyzInertial;
      | uvwGround;
      | attitude;
      | pqr;
      | airspeed;
      | groundSpeed;
      | courseAngle]
  Aircraft States : Inport
  Add2 : Sum
  Airspeed noise : RandomNumber  SampleTime=0.1
  Gain1 : Gain  Gain=sensorNoiseFlag
  Mux : Mux  Inputs=6
  Select Va (idx = 13) : Selector  InputPortWidth=15  IndexOptions=Index vector (dialog)  Indices=13  OutputSizes=1
  Select phi (idx = 7) : Selector  InputPortWidth=15  IndexOptions=Index vector (dialog)  Indices=7  OutputSizes=1
  Select psi (idx = 9) : Selector  InputPortWidth=15  IndexOptions=Index vector (dialog)  Indices=9  OutputSizes=1
  Select r (idx = 11) : Selector  InputPortWidth=15  IndexOptions=Index vector (dialog)  Indices=11  OutputSizes=1
  Select r (idx = 12) : Selector  InputPortWidth=15  IndexOptions=Index vector (dialog)  Indices=12  OutputSizes=1
  Select theta (idx = 8) : Selector  InputPortWidth=15  IndexOptions=Index vector (dialog)  Indices=8  OutputSizes=1
  u : Outport
  wires:
  Aircraft States/1 -> Select psi (idx = 9)/1, Select theta (idx = 8)/1, Select phi (idx = 7)/1, Select r (idx = 12)/1, Select r (idx = 11)/1, Select Va (idx = 13)/1
  Mux/1 -> u/1
  Select r (idx = 11)/1 -> Mux/2
  Select Va (idx = 13)/1 -> Add2/2
  Select r (idx = 12)/1 -> Mux/3
  Select phi (idx = 7)/1 -> Mux/4
  Select theta (idx = 8)/1 -> Mux/5
  Select psi (idx = 9)/1 -> Mux/6  "selPsi"
  Gain1/1 -> Add2/1
  Airspeed noise/1 -> Gain1/1
  Add2/1 -> Mux/1

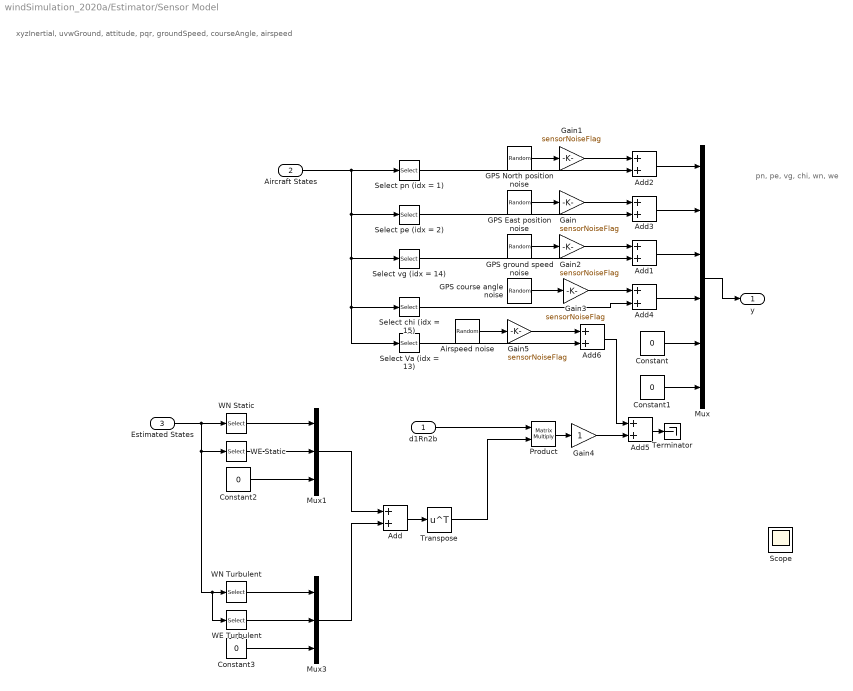
== system windSimulation_2020a/Estimator/Sensor Model ==
  note: pn, pe, vg, chi, wn, we
  note: xyzInertial, uvwGround, attitude, pqr, groundSpeed, courseAngle, airspeed
  d1Rn2b : Inport
  Aircraft States : Inport  Port=2
  Estimated States : Inport  Port=3
  Add{,1..6} (7 alike) : Sum
  Airspeed noise : RandomNumber  Variance=var.airspeed_mps  SampleTime=dt
  Constant{,1..3} (4 alike) : Constant  Value=0
  GPS East position noise : RandomNumber  Variance=var.position_m  SampleTime=dt
  GPS North position noise : RandomNumber  Variance=var.position_m  SampleTime=dt
  GPS course angle noise : RandomNumber  Variance=var.attitude_rad * 3  SampleTime=dt
  GPS ground speed noise : RandomNumber  Variance=var.velocityGps_mps  SampleTime=dt
  Gain{,1..3,5} (5 alike) : Gain  Gain=sensorNoiseFlag
  Gain4 : Gain
  Mux : Mux  Inputs=6
  Mux1 : Mux  Inputs=3
  Mux3 : Mux  Inputs=3
  Product : Product  Multiplication=Matrix(*)
  Scope : Scope
  Select Va (idx = 13) : Selector  InputPortWidth=nStates  IndexOptions=Index vector (dialog)  Indices=13  OutputSizes=1
  Select chi (idx = 15) : Selector  InputPortWidth=nStates  IndexOptions=Index vector (dialog)  Indices=15  OutputSizes=1
  Select pe (idx = 2) : Selector  InputPortWidth=nStates  IndexOptions=Index vector (dialog)  Indices=2  OutputSizes=1
  Select pn (idx = 1) : Selector  InputPortWidth=nStates  IndexOptions=Index vector (dialog)  Indices=1  OutputSizes=1
  Select vg (idx = 14) : Selector  InputPortWidth=nStates  IndexOptions=Index vector (dialog)  Indices=14  OutputSizes=1
  Terminator : Terminator
  Transpose : Math  Operator=transpose  SaturateOnIntegerOverflow=on
  WE Static : Selector  InputPortWidth=nEstStates  IndexOptions=Index vector (dialog)  Indices=6  OutputSizes=1
  WE Turbulent : Selector  InputPortWidth=nEstStates  IndexOptions=Index vector (dialog)  Indices=8  OutputSizes=1
  WN Static : Selector  InputPortWidth=nEstStates  IndexOptions=Index vector (dialog)  Indices=5  OutputSizes=1
  WN Turbulent : Selector  InputPortWidth=nEstStates  IndexOptions=Index vector (dialog)  Indices=7  OutputSizes=1
  y : Outport
  wires:
  Aircraft States/1 -> Select Va (idx = 13)/1, Select chi (idx = 15)/1, Select vg (idx = 14)/1, Select pe (idx = 2)/1, Select pn (idx = 1)/1
  Mux/1 -> y/1
  GPS ground speed noise/1 -> Gain2/1
  Add2/1 -> Mux/1
  Select pn (idx = 1)/1 -> Add2/2
  GPS North position noise/1 -> Gain1/1
  Add3/1 -> Mux/2
  GPS East position noise/1 -> Gain/1
  Select pe (idx = 2)/1 -> Add3/2
  GPS course angle noise/1 -> Gain3/1
  Add4/1 -> Mux/4
  Add1/1 -> Mux/3
  WN Static/1 -> Mux1/1
  WE Static/1 -> Mux1/2
  Gain/1 -> Add3/1
  Gain1/1 -> Add2/1
  Gain2/1 -> Add1/1
  Gain3/1 -> Add4/1
  Select vg (idx = 14)/1 -> Add1/2
  Select chi (idx = 15)/1 -> Add4/2
  Estimated States/1 -> WE Turbulent/1, WN Turbulent/1, WE Static/1, WN Static/1
  WN Turbulent/1 -> Mux3/1
  WE Turbulent/1 -> Mux3/2
  Constant/1 -> Mux/5
  Constant1/1 -> Mux/6
  Constant2/1 -> Mux1/3
  Constant3/1 -> Mux3/3
  Mux1/1 -> Add/1
  Mux3/1 -> Add/2
  Add/1 -> Transpose/1
  Transpose/1 -> Product/2
  Product/1 -> Gain4/1
  d1Rn2b/1 -> Product/1
  Airspeed noise/1 -> Gain5/1
  Gain5/1 -> Add6/1
  Select Va (idx = 13)/1 -> Add6/2
  Gain4/1 -> Add5/2
  Add5/1 -> Terminator/1
  Add6/1 -> Add5/1

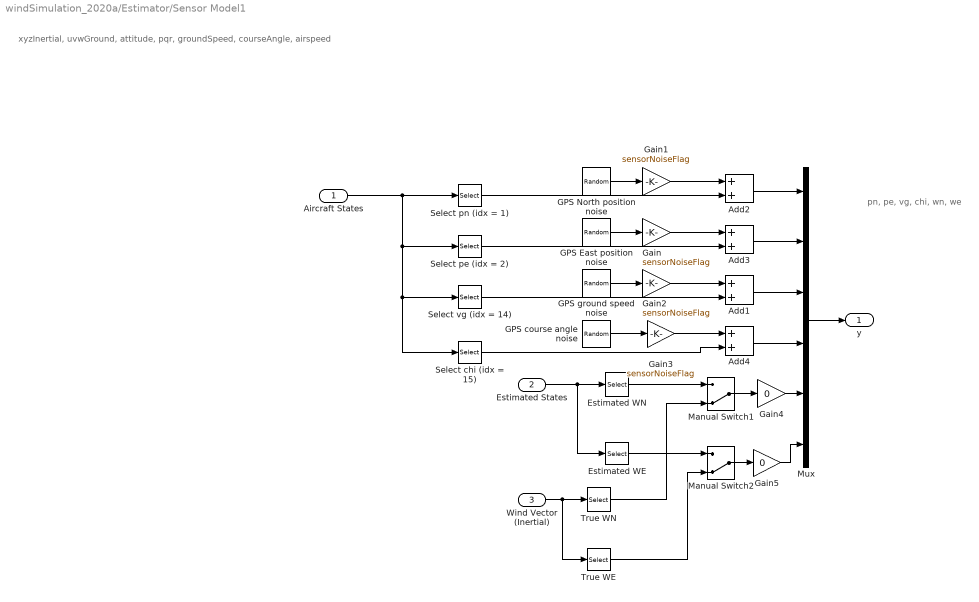
== system windSimulation_2020a/Estimator/Sensor Model1 ==
  note: pn, pe, vg, chi, wn, we
  note: xyzInertial, uvwGround, attitude, pqr, groundSpeed, courseAngle, airspeed
  Aircraft States : Inport
  Estimated States : Inport  Port=2
  Wind Vector (Inertial) : Inport  Port=3
  Add{1..4} (4 alike) : Sum
  Estimated WE : Selector  InputPortWidth=6  IndexOptions=Index vector (dialog)  Indices=6  OutputSizes=1
  Estimated WN : Selector  InputPortWidth=6  IndexOptions=Index vector (dialog)  Indices=5  OutputSizes=1
  GPS East position noise : RandomNumber  SampleTime=0.1
  GPS North position noise : RandomNumber  SampleTime=0.1
  GPS course angle noise : RandomNumber  SampleTime=0.1
  GPS ground speed noise : RandomNumber  SampleTime=0.1
  Gain{,1..3} (4 alike) : Gain  Gain=sensorNoiseFlag
  Gain4 : Gain  Gain=0
  Gain5 : Gain  Gain=0
  Manual Switch1 : ManualSwitch  CurrentSetting=0
  Manual Switch2 : ManualSwitch  CurrentSetting=0
  Mux : Mux  Inputs=6
  Select chi (idx = 15) : Selector  InputPortWidth=15  IndexOptions=Index vector (dialog)  Indices=15  OutputSizes=1
  Select pe (idx = 2) : Selector  InputPortWidth=15  IndexOptions=Index vector (dialog)  Indices=2  OutputSizes=1
  Select pn (idx = 1) : Selector  InputPortWidth=15  IndexOptions=Index vector (dialog)  Indices=1  OutputSizes=1
  Select vg (idx = 14) : Selector  InputPortWidth=15  IndexOptions=Index vector (dialog)  Indices=14  OutputSizes=1
  True WE : Selector  InputPortWidth=6  IndexOptions=Index vector (dialog)  Indices=6  OutputSizes=1
  True WN : Selector  InputPortWidth=6  IndexOptions=Index vector (dialog)  Indices=5  OutputSizes=1
  y : Outport
  wires:
  Aircraft States/1 -> Select chi (idx = 15)/1, Select vg (idx = 14)/1, Select pe (idx = 2)/1, Select pn (idx = 1)/1
  Mux/1 -> y/1
  GPS ground speed noise/1 -> Gain2/1
  Add2/1 -> Mux/1
  Select pn (idx = 1)/1 -> Add2/2
  GPS North position noise/1 -> Gain1/1
  Add3/1 -> Mux/2
  GPS East position noise/1 -> Gain/1
  Select pe (idx = 2)/1 -> Add3/2
  GPS course angle noise/1 -> Gain3/1
  Add4/1 -> Mux/4
  Add1/1 -> Mux/3
  Estimated States/1 -> Estimated WE/1, Estimated WN/1
  Estimated WN/1 -> Manual Switch1/1
  Estimated WE/1 -> Manual Switch2/1
  Gain/1 -> Add3/1
  Gain1/1 -> Add2/1
  Gain2/1 -> Add1/1
  Gain3/1 -> Add4/1
  Select vg (idx = 14)/1 -> Add1/2
  Select chi (idx = 15)/1 -> Add4/2
  Manual Switch1/1 -> Gain4/1
  Manual Switch2/1 -> Gain5/1
  Wind Vector (Inertial)/1 -> True WE/1, True WN/1
  True WN/1 -> Manual Switch1/2
  True WE/1 -> Manual Switch2/2
  Gain4/1 -> Mux/5
  Gain5/1 -> Mux/6

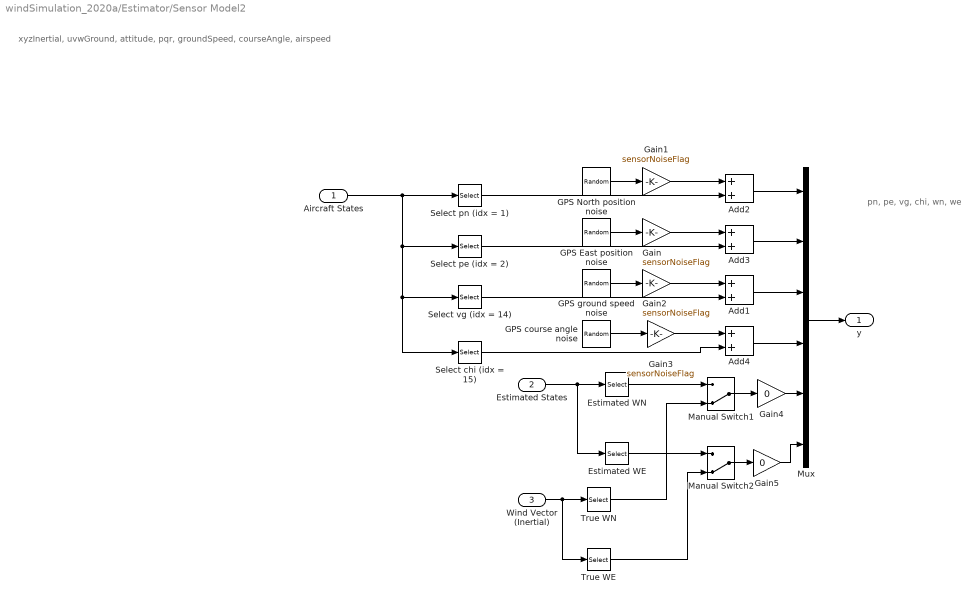
== system windSimulation_2020a/Estimator/Sensor Model2 ==
  note: pn, pe, vg, chi, wn, we
  note: xyzInertial, uvwGround, attitude, pqr, groundSpeed, courseAngle, airspeed
  Aircraft States : Inport
  Estimated States : Inport  Port=2
  Wind Vector (Inertial) : Inport  Port=3
  Add{1..4} (4 alike) : Sum
  Estimated WE : Selector  InputPortWidth=6  IndexOptions=Index vector (dialog)  Indices=6  OutputSizes=1
  Estimated WN : Selector  InputPortWidth=6  IndexOptions=Index vector (dialog)  Indices=5  OutputSizes=1
  GPS East position noise : RandomNumber  SampleTime=0.1
  GPS North position noise : RandomNumber  SampleTime=0.1
  GPS course angle noise : RandomNumber  SampleTime=0.1
  GPS ground speed noise : RandomNumber  SampleTime=0.1
  Gain{,1..3} (4 alike) : Gain  Gain=sensorNoiseFlag
  Gain4 : Gain  Gain=0
  Gain5 : Gain  Gain=0
  Manual Switch1 : ManualSwitch  CurrentSetting=0
  Manual Switch2 : ManualSwitch  CurrentSetting=0
  Mux : Mux  Inputs=6
  Select chi (idx = 15) : Selector  InputPortWidth=15  IndexOptions=Index vector (dialog)  Indices=15  OutputSizes=1
  Select pe (idx = 2) : Selector  InputPortWidth=15  IndexOptions=Index vector (dialog)  Indices=2  OutputSizes=1
  Select pn (idx = 1) : Selector  InputPortWidth=15  IndexOptions=Index vector (dialog)  Indices=1  OutputSizes=1
  Select vg (idx = 14) : Selector  InputPortWidth=15  IndexOptions=Index vector (dialog)  Indices=14  OutputSizes=1
  True WE : Selector  InputPortWidth=6  IndexOptions=Index vector (dialog)  Indices=6  OutputSizes=1
  True WN : Selector  InputPortWidth=6  IndexOptions=Index vector (dialog)  Indices=5  OutputSizes=1
  y : Outport
  wires:
  Aircraft States/1 -> Select chi (idx = 15)/1, Select vg (idx = 14)/1, Select pe (idx = 2)/1, Select pn (idx = 1)/1
  Mux/1 -> y/1
  GPS ground speed noise/1 -> Gain2/1
  Add2/1 -> Mux/1
  Select pn (idx = 1)/1 -> Add2/2
  GPS North position noise/1 -> Gain1/1
  Add3/1 -> Mux/2
  GPS East position noise/1 -> Gain/1
  Select pe (idx = 2)/1 -> Add3/2
  GPS course angle noise/1 -> Gain3/1
  Add4/1 -> Mux/4
  Add1/1 -> Mux/3
  Estimated States/1 -> Estimated WE/1, Estimated WN/1
  Estimated WN/1 -> Manual Switch1/1
  Estimated WE/1 -> Manual Switch2/1
  Gain/1 -> Add3/1
  Gain1/1 -> Add2/1
  Gain2/1 -> Add1/1
  Gain3/1 -> Add4/1
  Select vg (idx = 14)/1 -> Add1/2
  Select chi (idx = 15)/1 -> Add4/2
  Manual Switch1/1 -> Gain4/1
  Manual Switch2/1 -> Gain5/1
  Wind Vector (Inertial)/1 -> True WE/1, True WN/1
  True WN/1 -> Manual Switch1/2
  True WE/1 -> Manual Switch2/2
  Gain4/1 -> Mux/5
  Gain5/1 -> Mux/6

== system windSimulation_2020a/Subsystem1/Get ground speed and course angle ==
  Ground Velocity : Inport
  Atan2 : Trigonometry  Operator=atan2
  Dot Product : DotProduct  InputSameDT=on  OutDataTypeStr=Inherit: Inherit via internal rule
  Selector : Selector  InputPortWidth=3  IndexOptions=Index vector (dialog)  Indices=2  OutputSizes=1
  Selector1 : Selector  InputPortWidth=3  IndexOptions=Index vector (dialog)  Indices=1  OutputSizes=1
  Sqrt : Sqrt  SaturateOnIntegerOverflow=on
  Ground Speed : Outport
  Course Angle : Outport  Port=2
  wires:
  Selector1/1 -> Atan2/2
  Selector/1 -> Atan2/1
  Ground Velocity/1 -> Dot Product/2, Dot Product/1, Selector1/1, Selector/1
  Atan2/1 -> Course Angle/1  "trueCourseAngle"
  Dot Product/1 -> Sqrt/1
  Sqrt/1 -> Ground Speed/1

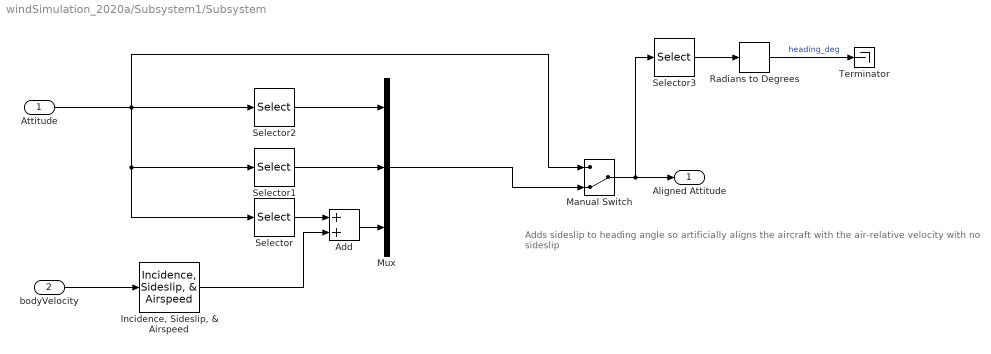
== system windSimulation_2020a/Subsystem1/Subsystem ==
  note: Adds sideslip to heading angle so artificially aligns the aircraft with the air-relative velocity with no sideslip
  Attitude : Inport
  bodyVelocity : Inport  Port=2
  Add : Sum
  "Incidence, Sideslip, & Airspeed" : aerolibasang/Incidence, Sideslip, & Airspeed
  Manual Switch : ManualSwitch  CurrentSetting=0
  Mux : Mux  Inputs=3
  Radians to Degrees : simulink_extras/Transformations/Radians to Degrees
  Selector : Selector  InputPortWidth=3  IndexOptions=Index vector (dialog)  Indices=3  OutputSizes=1
  Selector1 : Selector  InputPortWidth=3  IndexOptions=Index vector (dialog)  Indices=2  OutputSizes=1
  Selector2 : Selector  InputPortWidth=3  IndexOptions=Index vector (dialog)  Indices=1  OutputSizes=1
  Selector3 : Selector  InputPortWidth=3  IndexOptions=Index vector (dialog)  Indices=3  OutputSizes=1
  Terminator : Terminator
  Aligned Attitude : Outport
  wires:
  bodyVelocity/1 -> "Incidence, Sideslip, & Airspeed"/1
  Attitude/1 -> Manual Switch/1, Selector1/1, Selector/1, Selector2/1
  Mux/1 -> Manual Switch/2
  Add/1 -> Mux/3
  "Incidence, Sideslip, & Airspeed"/2 -> Add/2
  Selector/1 -> Add/1
  Selector1/1 -> Mux/2
  Selector2/1 -> Mux/1
  Manual Switch/1 -> Selector3/1, Aligned Attitude/1
  Selector3/1 -> Radians to Degrees/1
  Radians to Degrees/1 -> Terminator/1  "heading_deg"

== matlab function windSimulation_2020a/Estimator/MATLAB Function1 ==
  data: mu_km_km input; mu_k_k output; Sig_km_km input; u_km input; y_k input; Q input; R input; dt input; Sig_k_k output
%% Unscented Kalman Filter
function [mu_k_k,Sig_k_k] = UKF(mu_km_km, Sig_km_km, u_km, y_k, Q, R, dt)
%     global xdim; global ydim;
    xdim = size(mu_km_km,1); ydim = size(y_k,1);
    % predict step
    % mu_km_km is of size (n,1), prior_points is of size (n,2n+1), weights is of size (2n+1,1)
    [prior_points, w0, wi] = UT(mu_km_km, Sig_km_km);
    pred_points = prior_points;
    for i = 1:2*xdim+1
        pred_points(:,i) = dynamics(prior_points(:,i), u_km, dt);
    end
    [mu_k_km, Sig_k_km] = UTinv(pred_points, w0, wi, Q);
    
    % update step
    [update_points, w0, wi] = UT(mu_k_km, Sig_k_km); % update_points and pred_points same?
%     update_points = pred_points;
    y_true = zeros(ydim,2*xdim+1);
    y_est = zeros(ydim,1);
    for i = 1:size(update_points,2)
        y_true(:,i) = getMeasurementModel(update_points(:,i),u_km);
    end
    y_est = w0*y_true(:,1) + wi*sum(y_true(:,2:end),2);
    Cov_Y = zeros(ydim,ydim);
    Cov_XY = zeros(xdim,ydim);
    for i = 1:2*xdim+1
        if i == 1
            wt_i = w0;
        else
            wt_i = wi;
        end
        Cov_Y = Cov_Y + wt_i*(y_true(:,i)-y_est)*(y_true(:,i)-y_est)';
        Cov_XY = Cov_XY + wt_i*(update_points(:,i)-mu_k_km)*(y_true(:,i)-y_est)';
    end
    Cov_Y = Cov_Y + R;
    mu_k_k = mu_k_km + Cov_XY*inv(Cov_Y)*(y_k - y_est);
    Sig_k_k = Sig_k_km - Cov_XY*inv(Cov_Y)*Cov_XY'; 
end

%% Helper functions for UKF
% mu_km_km is of size (xdim,1), prior_points is of size (xdim,2n+1)
function [prior_points, w0, wi] = UT(mu, Sig)
    lambda = 2;
    xdim = size(mu,1);
    prior_points = zeros(xdim, 2*xdim+1);
    % weights
    w0 = lambda/(lambda+xdim);
    wi = 1/(2*(lambda+xdim));
    % 0 point
    prior_points(:,1) = mu;
    matrix_sqr_root = real(sqrtm((lambda+xdim)*Sig));
    for i = 1:xdim
        % ith point
        prior_points(:,1+i) = mu + matrix_sqr_root(:,i);
        % i + nth point
        prior_points(:,1+i+xdim) = mu - matrix_sqr_root(:,i);
    end
end

% points is of size (n,2n+1)
function [mu, Sig] = UTinv(points, w0, wi, Q)
%     global xdim;
    xdim = size(points(:,1),1);
    n = xdim;
    mu = zeros(n,1);
    Sig = zeros(n,n);
    mu = w0*points(:,1) + wi*sum(points(:,2:end),2);
    for i = 1:2*n+1
        if i == 1
            Sig = Sig + w0*(points(:,i) - mu)*(points(:,i) - mu)';
        else
            Sig = Sig + wi*(points(:,i) - mu)*(points(:,i) - mu)';
        end
    end
    Sig = Sig + Q;
end

== matlab function windSimulation_2020a/Estimator/MATLAB Function2 ==
  data: mu_km_km input; mu_k_k output; Sig_km_km input; u_km input; y_k input; Q input; R input; dt input; num_particles input; Sig_k_k output; rand_norm_nums input; rand_uniform_nums input
%% Particle filter
function [mu_k_k, Sig_k_k] = particle_filter(mu_km_km, Sig_km_km, u_km, y_k, Q, R, dt, num_particles, rand_norm_nums, rand_uniform_nums)
%     num_particles = 100;
    % sample particles
    prior_points = make_particles(mu_km_km,Sig_km_km,num_particles, rand_norm_nums);    
    % predict step
    pred_points = prior_points;
    unnorm_weights = zeros(num_particles);
    inv_R = inv(R); % precalculate just once
    for i = 1:num_particles
        % predict points
        pred_points(:,i) = dynamics(prior_points(:,i), u_km, dt);
        % update weights
        unnorm_weights(i) = gaussian_pdf(y_k, getMeasurementModel(pred_points(:,i), u_km), inv_R);
    end
    norm_weights = unnorm_weights/sum(unnorm_weights);
    % resample particles 
    post_points = resample_particles(norm_weights, pred_points, rand_uniform_nums);
    [mu_k_k, Sig_k_k] = get_mu_sig_from_particles(post_points); 
    
%     mu_k_k = mu_km_km;
%     Sig_k_k = Sig_km_km;
%     [mu_k_k, Sig_k_k] = get_mu_sig_from_particles(pred_points);
end

%% Helper functions for particle filter
function particles = make_particles(mu,Sig,num_particles, rand_norm_nums)
    % create 1000 particles
    xdim = size(mu,1);
%     particles = zeros(xdim, num_particles); 
%     particles = repmat(mu,1,num_particles) + chol(Sig)*randn(xdim,num_particles);
    rand_norm_nums = reshape(rand_norm_nums, xdim, num_particles);
    particles = repmat(mu,1,num_particles) + real(sqrtm(Sig))*rand_norm_nums;
end

function [mu,Sig] = get_mu_sig_from_particles(particles)
    mu = mean(particles,2);
    Sig = cov(particles');
    xdim = size(mu,1);
    Sig = Sig(1:xdim,1:xdim);
end

% function new_particles = resample_particles_prob_fun(weights, particles)
%     % points ~(xdim, num_particles)
%     % weights ~(num_particles,1)
%     num_particles = size(particles,2);
%     % Get new indices
%     inds = randsample(1:num_particles, num_particles, true, weights);
%     new_particles = particles(:,inds);
% end

function new_particles = resample_particles(weights, particles, rand_uniform_nums)
    % points ~(xdim, num_particles)
    % weights ~(num_particles,1)
%     global xdim;
    xdim = size(particles,1);
    num_particles = size(particles,2);
    new_particles = zeros(xdim, num_particles);
    % create cum_weights vector
    cum_weights = zeros(num_particles,1);
    cum_weights(1) = weights(1);
    for j = 2:num_particles
        cum_weights(j) = cum_weights(j-1) + weights(j);
    end
    for j = 1:num_particles
%         s_j = rand();
        s_j = rand_uniform_nums(j);
        first_higher_index = find(cum_weights>s_j,1);
        new_particles(:,j) = particles(:,first_higher_index);
    end
end

function likelihood = gaussian_pdf(x, mu, inv_Sig)
    resid = x - mu;
    likelihood = exp(-0.5*resid'*inv_Sig*resid);    
end

== matlab function windSimulation_2020a/Estimator/MATLAB Function ==
  data: mu_k input; mu_kp output; Sig_k input; u_k input; y_kp input; Q input; R input; dt input; Sig_kp output
function [mu_kp, Sig_kp] = extendedKalmanFilter(mu_k, Sig_k, u_k, y_kp, Q, R, dt)
    % Prediction step
    A = getDynamicsJacobian(mu_k, u_k, dt);
    mu_pred = dynamics(mu_k, u_k, dt);
    Sig_pred = Sig_k + dt*(A*Sig_k + Sig_k*transpose(A) + Q);

    % Using state transition dynamics/matrix
%     A        = getStateTransitionDynamics(mu_k, u_k, dt);
%     mu_pred  = transitionDynamics(mu_k, u_k, dt);
%     Sig_pred = A*Sig_k*A' + Q;

%% TEST TO GET TURBULENCE ESTIMATES
    % Prediction step
%     A = getDynamicsJacobianTest(mu_k, u_k, dt);
%     mu_pred  = transitionDynamicsTest(mu_k, u_k, dt);
%     Sig_pred = Sig_k + dt*(A*Sig_k + Sig_k*transpose(A) + Q);


%%
    % Update step
    C = getMeasurementJacobian(mu_pred, u_k);
    ybar = y_kp - getMeasurementModel(mu_pred, u_k);
    K = Sig_pred*C'/(C*Sig_pred*C' + R); % Kalman gain
    mu_kp = mu_pred + K*ybar;
    Sig_kp = Sig_pred - K*C*Sig_pred;
    
%     coder.extrinsic('obsv');
%     O = obsv(A, C);
%     rank(O)
end
